simulink model "IEEE14_case"  (R2024b)
settings: Solver=FixedStepAuto  StartTime=0  StopTime=2  FixedStep=1e-7  RelTol=1e-3
values from neighbouring files (symbols this model uses):
  GFL_15_Bva = 0.009    [IEEE14_parameters.m]
  GFL_15_C_bus_pu = 7.179419    [IEEE14_parameters.m]
  GFL_15_f0 = 60    [IEEE14_parameters.m]
  GFL_15_I_id = 691.26967    [IEEE14_parameters.m]
  GFL_15_I_iq = 691.26967    [IEEE14_parameters.m]
  GFL_15_I_od = 45.2207    [IEEE14_parameters.m]
  GFL_15_I_oq = 45.2207    [IEEE14_parameters.m]
  GFL_15_I_pll = 0.78    [IEEE14_parameters.m]
  GFL_15_Kdi = 0.09    [IEEE14_parameters.m]
  GFL_15_Kdo = 0.9    [IEEE14_parameters.m]
  GFL_15_Kqi = 0.09    [IEEE14_parameters.m]
  GFL_15_Kqo = 0.9    [IEEE14_parameters.m]
  GFL_15_Lg_pu = 0.631447    [IEEE14_parameters.m]
  GFL_15_mode = 1    [IEEE14_parameters.m]
  GFL_15_P_id = 3.7166    [IEEE14_parameters.m]
  GFL_15_P_iq = 3.7166    [IEEE14_parameters.m]
  GFL_15_P_od = 0.4798    [IEEE14_parameters.m]
  GFL_15_P_oq = 0.4798    [IEEE14_parameters.m]
  GFL_15_P_pll = 290.42    [IEEE14_parameters.m]
  GFL_15_Qe_ref = 0.2    [IEEE14_parameters.m]
  GFL_15_Rg_pu = 0.024016    [IEEE14_parameters.m]
  GFL_15_Sbase = 1.000000e+4    (= 10000)    [IEEE14_parameters.m]
  GFL_15_Tdi = 0.01    [IEEE14_parameters.m]
  GFL_15_Tdo = 0.2    [IEEE14_parameters.m]
  GFL_15_Tqi = 0.01    [IEEE14_parameters.m]
  GFL_15_Tqo = 0.2    [IEEE14_parameters.m]
  GFL_15_Vbase = 380    [IEEE14_parameters.m]
  GFL_15_Vdc_ref = 1.011475    [IEEE14_parameters.m]
  GFL_15_Vdcbase = 700    [IEEE14_parameters.m]
  GFL_15_vq_ref = 0    [IEEE14_parameters.m]
  GFL_16_Bva = 0.002    [IEEE14_parameters.m]
  GFL_16_C_bus_pu = 7.179419    [IEEE14_parameters.m]
  GFL_16_f0 = 60    [IEEE14_parameters.m]
  GFL_16_I_id = 691.26967    [IEEE14_parameters.m]
  GFL_16_I_iq = 691.26967    [IEEE14_parameters.m]
  GFL_16_I_od = 45.2207    [IEEE14_parameters.m]
  GFL_16_I_oq = 45.2207    [IEEE14_parameters.m]
  GFL_16_I_pll = 0.78    [IEEE14_parameters.m]
  GFL_16_Kdi = 0.05    [IEEE14_parameters.m]
  GFL_16_Kdo = 0.5    [IEEE14_parameters.m]
  GFL_16_Kqi = 0.05    [IEEE14_parameters.m]
  GFL_16_Kqo = 0.5    [IEEE14_parameters.m]
  GFL_16_Lg_pu = 0.631447    [IEEE14_parameters.m]
  GFL_16_mode = 1    [IEEE14_parameters.m]
  GFL_16_P_id = 3.7166    [IEEE14_parameters.m]
  GFL_16_P_iq = 3.7166    [IEEE14_parameters.m]
  GFL_16_P_od = 0.4798    [IEEE14_parameters.m]
  GFL_16_P_oq = 0.4798    [IEEE14_parameters.m]
  GFL_16_P_pll = 290.42    [IEEE14_parameters.m]
  GFL_16_Qe_ref = 0.2    [IEEE14_parameters.m]
  GFL_16_Rg_pu = 0.024016    [IEEE14_parameters.m]
  GFL_16_Sbase = 1.000000e+4    (= 10000)    [IEEE14_parameters.m]
  GFL_16_Tdi = 0.01    [IEEE14_parameters.m]
  GFL_16_Tdo = 0.2    [IEEE14_parameters.m]
  GFL_16_Tqi = 0.01    [IEEE14_parameters.m]
  GFL_16_Tqo = 0.2    [IEEE14_parameters.m]
  GFL_16_Vbase = 380    [IEEE14_parameters.m]
  GFL_16_Vdc_ref = 1.01144    [IEEE14_parameters.m]
  GFL_16_Vdcbase = 700    [IEEE14_parameters.m]
  GFL_16_vq_ref = 0    [IEEE14_parameters.m]
  GFL_17_Bva = 0.002    [IEEE14_parameters.m]
  GFL_17_C_bus_pu = 7.179419    [IEEE14_parameters.m]
  GFL_17_f0 = 60    [IEEE14_parameters.m]
  GFL_17_I_id = 691.26967    [IEEE14_parameters.m]
  GFL_17_I_iq = 691.26967    [IEEE14_parameters.m]
  GFL_17_I_od = 45.2207    [IEEE14_parameters.m]
  GFL_17_I_oq = 45.2207    [IEEE14_parameters.m]
  GFL_17_I_pll = 0.78    [IEEE14_parameters.m]
  GFL_17_Kdi = 0.05    [IEEE14_parameters.m]
  GFL_17_Kdo = 0.5    [IEEE14_parameters.m]
  GFL_17_Kqi = 0.05    [IEEE14_parameters.m]
  GFL_17_Kqo = 0.5    [IEEE14_parameters.m]
  GFL_17_Lg_pu = 0.631447    [IEEE14_parameters.m]
  GFL_17_mode = 1    [IEEE14_parameters.m]
  GFL_17_P_id = 3.7166    [IEEE14_parameters.m]
  GFL_17_P_iq = 3.7166    [IEEE14_parameters.m]
  GFL_17_P_od = 0.4798    [IEEE14_parameters.m]
  GFL_17_P_oq = 0.4798    [IEEE14_parameters.m]
  GFL_17_P_pll = 290.42    [IEEE14_parameters.m]
  GFL_17_Qe_ref = 0.2    [IEEE14_parameters.m]
  GFL_17_Rg_pu = 0.024016    [IEEE14_parameters.m]
  GFL_17_Sbase = 1.000000e+4    (= 10000)    [IEEE14_parameters.m]
  GFL_17_Tdi = 0.01    [IEEE14_parameters.m]
  GFL_17_Tdo = 0.2    [IEEE14_parameters.m]
  GFL_17_Tqi = 0.01    [IEEE14_parameters.m]
  GFL_17_Tqo = 0.2    [IEEE14_parameters.m]
  GFL_17_Vbase = 380    [IEEE14_parameters.m]
  GFL_17_Vdc_ref = 1.011632    [IEEE14_parameters.m]
  GFL_17_Vdcbase = 700    [IEEE14_parameters.m]
  GFL_17_vq_ref = 0    [IEEE14_parameters.m]
  GFL_18_Bva = 0.002    [IEEE14_parameters.m]
  GFL_18_C_bus_pu = 7.179419    [IEEE14_parameters.m]
  GFL_18_f0 = 60    [IEEE14_parameters.m]
  GFL_18_I_id = 691.26967    [IEEE14_parameters.m]
  GFL_18_I_iq = 691.26967    [IEEE14_parameters.m]
  GFL_18_I_od = 45.2207    [IEEE14_parameters.m]
  GFL_18_I_oq = 45.2207    [IEEE14_parameters.m]
  GFL_18_I_pll = 0.78    [IEEE14_parameters.m]
  GFL_18_Kdi = 0.05    [IEEE14_parameters.m]
  GFL_18_Kdo = 0.5    [IEEE14_parameters.m]
  GFL_18_Kqi = 0.05    [IEEE14_parameters.m]
  GFL_18_Kqo = 0.5    [IEEE14_parameters.m]
  GFL_18_Lg_pu = 0.631447    [IEEE14_parameters.m]
  GFL_18_mode = 1    [IEEE14_parameters.m]
  GFL_18_P_id = 3.7166    [IEEE14_parameters.m]
  GFL_18_P_iq = 3.7166    [IEEE14_parameters.m]
  GFL_18_P_od = 0.4798    [IEEE14_parameters.m]
  GFL_18_P_oq = 0.4798    [IEEE14_parameters.m]
  GFL_18_P_pll = 290.42    [IEEE14_parameters.m]
  GFL_18_Qe_ref = 0.2    [IEEE14_parameters.m]
  GFL_18_Rg_pu = 0.024016    [IEEE14_parameters.m]
  GFL_18_Sbase = 1.000000e+4    (= 10000)    [IEEE14_parameters.m]
  GFL_18_Tdi = 0.01    [IEEE14_parameters.m]
  GFL_18_Tdo = 0.2    [IEEE14_parameters.m]
  GFL_18_Tqi = 0.01    [IEEE14_parameters.m]
  GFL_18_Tqo = 0.2    [IEEE14_parameters.m]
  GFL_18_Vbase = 380    [IEEE14_parameters.m]
  GFL_18_Vdc_ref = 1.011572    [IEEE14_parameters.m]
  GFL_18_Vdcbase = 700    [IEEE14_parameters.m]
  GFL_18_vq_ref = 0    [IEEE14_parameters.m]
  ... (+180 more)
(part 15 of 25)

== system IEEE14_case/GFL_18/d_i_gq_GFL_18_block ==
  note: d_i_gq_GFL_18 in case14gfl
      | $\frac{2\,\pi \,\mathrm{Sbase}\,f_{0}\,\left(\Phi _{\mathrm{gd},\mathrm{GFL},18}+P_{\mathrm{iq}}\,\left(\mathrm{Iqv}_{\mathrm{GFL},18}+\Phi _{\mathrm{gc},\mathrm{GFL},18}-i_{\mathrm{gq},\mathrm{GFL},18}-P_{\mathrm{oq}}\,\left(\mathrm{Qe}_{\mathrm{ref}}\,\mathrm{Sbase}+1.73205080756888\,\mathrm{Vbase}\,i_{\mathrm{gd},\mathrm{GFL},18}\,\left(v_{q,\mathrm{GFL},18}\,\cos\left(\theta _{\mathrm{pll},\mathrm{GFL},18}\right)+v_{d,\mathrm{GFL},18}\,\sin\left(\theta _{\mathrm{pll},\mathrm{GFL},18}\right)\right)+1.73205080756888\,\mathrm{Vbase}\,i_{\mathrm{gq},\mathrm{GFL},18}\,\left(v_{d,\mathrm{GFL},18}\,\cos\left(\theta _{\mathrm{pll},\mathrm{GFL},18}\right)-v_{q,\mathrm{GFL},18}\,\sin\left(\theta _{\mathrm{pll},\mathrm{GFL},18}\right)\right)\right)+\mathrm{Bva}\,\mathrm{Vbase}\,\left(v_{q,\mathrm{GFL},18}\,\cos\left(\theta _{\mathrm{pll},\mathrm{GFL},18}\right)+v_{d,\mathrm{GFL},18}\,\sin\left(\theta _{\mathrm{pll},\mathrm{GFL},18}\right)\right)\right)-\frac{\mathrm{Rg}_{\mathrm{pu}}\,{\mathrm{Vbase}}^2\,i_{\mathrm{gq},\mathrm{GFL},18}}{\mathrm{Sbase}}\right)}{\mathrm{Lg}_{\mathrm{pu}}\,{\mathrm{Vbase}}^2}$
      | Automatically generated on 2025-10-09 21:37:31 .
  Input_v_d_GFL_18_6f882 : Inport
  State_theta_pll_GFL_18_750f2 : Inport  Port=2
  Input_v_q_GFL_18_fb235 : Inport  Port=3
  State_theta_pll_GFL_18_9acfa : Inport  Port=4
  State_Iqv_GFL_18_30b1b : Inport  Port=5
  State_i_gd_GFL_18_52805 : Inport  Port=6
  Input_v_d_GFL_18_7a2d9 : Inport  Port=7
  State_theta_pll_GFL_18_d5076 : Inport  Port=8
  Input_v_q_GFL_18_2227f : Inport  Port=9
  State_theta_pll_GFL_18_46ba7 : Inport  Port=10
  State_i_gq_GFL_18_16534 : Inport  Port=11
  Input_v_d_GFL_18_2cf8e : Inport  Port=12
  State_theta_pll_GFL_18_ab8d9 : Inport  Port=13
  Input_v_q_GFL_18_563cc : Inport  Port=14
  State_theta_pll_GFL_18_cabe0 : Inport  Port=15
  State_Phi_gc_GFL_18_55584 : Inport  Port=16
  State_i_gq_GFL_18_9395d : Inport  Port=17
  State_Phi_gd_GFL_18_5fde0 : Inport  Port=18
  State_i_gq_GFL_18_b9a26 : Inport  Port=19
  Add_02e4d : Sum
  Add_19415 : Sum
  Add_1cbed : Sum
  Add_3289e : Sum
  Add_8a5df : Sum
  Add_efdee : Sum
  Constant_-1_893c0 : Constant  Value=-1
  Constant_1.73205080756888_7f0ab : Constant  Value=1.73205080756888
  Constant_1.73205080756888_dd0c5 : Constant  Value=1.73205080756888
  Constant_2.0_2560d : Constant  Value=2.0
  Constant_2.0_3ecfa : Constant  Value=2.0
  Constant_2.0_c0ff8 : Constant  Value=2.0
  Constant_Bva_65ebe : Constant  Value=Bva
  Constant_Lg_pu_8bb32 : Constant  Value=Lg_pu
  Constant_P_iq_7315b : Constant  Value=P_iq
  Constant_P_oq_2c47f : Constant  Value=P_oq
  Constant_Qe_ref_5f6bf : Constant  Value=Qe_ref
  Constant_Rg_pu_8e3e0 : Constant  Value=Rg_pu
  Constant_Sbase_2f81b : Constant  Value=Sbase
  Constant_Sbase_5e239 : Constant  Value=Sbase
  Constant_Sbase_94de3 : Constant  Value=Sbase
  Constant_Vbase_40973 : Constant  Value=Vbase
  Constant_Vbase_813da : Constant  Value=Vbase
  Constant_Vbase_8fd64 : Constant  Value=Vbase
  Constant_Vbase_ae26f : Constant  Value=Vbase
  Constant_Vbase_dbf74 : Constant  Value=Vbase
  Constant_f0_0d82f : Constant  Value=f0
  Constant_pi_8b980 : Constant  Value=pi
  Divide_20004 : Product  Inputs=*/
  Divide_d8df6 : Product  Inputs=*/
  MathFunc_cos_0de55 : Trigonometry  Operator=cos
  MathFunc_cos_104c8 : Trigonometry  Operator=cos
  MathFunc_cos_cc047 : Trigonometry  Operator=cos
  MathFunc_sin_52866 : Trigonometry
  MathFunc_sin_c83ee : Trigonometry
  MathFunc_sin_e5791 : Trigonometry
  Power_7e72b : Math  Operator=pow
  Power_8482d : Math  Operator=pow
  Product_00ff4 : Product
  Product_02cfb : Product
  Product_02fb3 : Product
  Product_04e48 : Product
  Product_17f28 : Product
  Product_1fcf9 : Product
  Product_354b2 : Product
  Product_380b4 : Product
  Product_38262 : Product
  Product_3b5ec : Product
  Product_3c14b : Product
  Product_4982c : Product
  Product_59f52 : Product
  Product_5af2a : Product
  Product_7f0f9 : Product
  Product_8339a : Product
  Product_99a53 : Product
  Product_acf9f : Product
  Product_afc64 : Product
  Product_b291c : Product
  Product_cbf79 : Product
  Product_ebe1d : Product
  Product_f803d : Product
  Product_fb3b2 : Product
  Product_fdbd3 : Product
  Subtract_3737a : Sum  Inputs=+-
  Subtract_401da : Sum  Inputs=+-
  Subtract_89c9e : Sum  Inputs=+-
  Subtract_e7562 : Sum  Inputs=+-
  Subtract_f2a58 : Sum  Inputs=+-
  Blockout_d_i_gq_GFL_18_699bd : Outport
  wires:
  State_theta_pll_GFL_18_d5076/1 -> MathFunc_sin_52866/1
  Constant_Vbase_ae26f/1 -> Product_38262/2
  State_theta_pll_GFL_18_46ba7/1 -> MathFunc_cos_cc047/1
  Constant_1.73205080756888_dd0c5/1 -> Product_38262/1
  Input_v_d_GFL_18_7a2d9/1 -> Product_3b5ec/1
  MathFunc_sin_52866/1 -> Product_3b5ec/2
  Product_acf9f/1 -> Add_efdee/2
  Input_v_q_GFL_18_2227f/1 -> Product_acf9f/1
  Constant_Sbase_5e239/1 -> Product_380b4/2
  MathFunc_cos_cc047/1 -> Product_acf9f/2
  Constant_Vbase_dbf74/1 -> Product_02fb3/2
  State_theta_pll_GFL_18_ab8d9/1 -> MathFunc_cos_0de55/1
  MathFunc_sin_e5791/1 -> Product_fb3b2/2
  State_theta_pll_GFL_18_cabe0/1 -> MathFunc_sin_e5791/1
  Constant_Qe_ref_5f6bf/1 -> Product_354b2/2
  State_theta_pll_GFL_18_750f2/1 -> MathFunc_sin_c83ee/1
  MathFunc_cos_104c8/1 -> Product_02cfb/2
  State_theta_pll_GFL_18_9acfa/1 -> MathFunc_cos_104c8/1
  Product_354b2/1 -> Product_380b4/1
  Constant_-1_893c0/1 -> Product_354b2/1
  Product_38262/1 -> Product_00ff4/1
  Product_3b5ec/1 -> Add_efdee/1
  State_i_gd_GFL_18_52805/1 -> Product_00ff4/2
  Product_02fb3/1 -> Product_f803d/1
  Constant_1.73205080756888_7f0ab/1 -> Product_02fb3/1
  Product_ebe1d/1 -> Subtract_f2a58/1
  Input_v_d_GFL_18_2cf8e/1 -> Product_ebe1d/1
  MathFunc_cos_0de55/1 -> Product_ebe1d/2
  Product_fb3b2/1 -> Subtract_f2a58/2
  Input_v_q_GFL_18_563cc/1 -> Product_fb3b2/1
  Product_59f52/1 -> Add_02e4d/1
  Input_v_d_GFL_18_6f882/1 -> Product_59f52/1
  MathFunc_sin_c83ee/1 -> Product_59f52/2
  Product_02cfb/1 -> Add_02e4d/2
  Constant_2.0_3ecfa/1 -> Power_7e72b/2
  Input_v_q_GFL_18_fb235/1 -> Product_02cfb/1
  Product_00ff4/1 -> Product_17f28/1
  Add_efdee/1 -> Product_17f28/2
  Subtract_f2a58/1 -> Product_fdbd3/2
  State_i_gq_GFL_18_16534/1 -> Product_f803d/2
  Constant_Sbase_2f81b/1 -> Product_5af2a/2
  Constant_2.0_c0ff8/1 -> Power_8482d/2
  Constant_Bva_65ebe/1 -> Product_7f0f9/1
  Constant_Vbase_8fd64/1 -> Power_8482d/1
  Product_7f0f9/1 -> Product_8339a/1
  Constant_Vbase_40973/1 -> Product_7f0f9/2
  Product_380b4/1 -> Subtract_89c9e/1
  Product_17f28/1 -> Subtract_89c9e/2
  Constant_2.0_2560d/1 -> Product_3c14b/1
  Product_f803d/1 -> Product_fdbd3/1
  Add_02e4d/1 -> Product_8339a/2
  Subtract_89c9e/1 -> Subtract_e7562/1
  Product_cbf79/1 -> Add_3289e/1
  Product_fdbd3/1 -> Subtract_e7562/2
  Power_8482d/1 -> Product_04e48/2
  Product_8339a/1 -> Add_8a5df/1
  Product_afc64/1 -> Add_1cbed/2
  Constant_P_oq_2c47f/1 -> Product_afc64/1
  State_Iqv_GFL_18_30b1b/1 -> Add_8a5df/2
  Subtract_e7562/1 -> Product_afc64/2
  Constant_Rg_pu_8e3e0/1 -> Product_04e48/1
  Add_19415/1 -> Subtract_3737a/1
  Add_8a5df/1 -> Add_1cbed/1
  Add_1cbed/1 -> Add_19415/1
  Product_5af2a/1 -> Product_b291c/1
  State_Phi_gc_GFL_18_55584/1 -> Add_19415/2
  State_i_gq_GFL_18_9395d/1 -> Subtract_3737a/2
  Divide_20004/1 -> Subtract_401da/2
  Constant_pi_8b980/1 -> Product_3c14b/2
  Constant_P_iq_7315b/1 -> Product_cbf79/1
  Subtract_3737a/1 -> Product_cbf79/2
  Product_04e48/1 -> Product_99a53/1
  State_i_gq_GFL_18_b9a26/1 -> Product_99a53/2
  Product_3c14b/1 -> Product_5af2a/1
  State_Phi_gd_GFL_18_5fde0/1 -> Add_3289e/2
  Product_99a53/1 -> Divide_20004/1
  Constant_Sbase_94de3/1 -> Divide_20004/2
  Constant_f0_0d82f/1 -> Product_b291c/2
  Add_3289e/1 -> Subtract_401da/1
  Constant_Vbase_813da/1 -> Power_7e72b/1
  Product_b291c/1 -> Product_4982c/1
  Subtract_401da/1 -> Product_4982c/2
  Constant_Lg_pu_8bb32/1 -> Product_1fcf9/1
  Power_7e72b/1 -> Product_1fcf9/2
  Product_4982c/1 -> Divide_d8df6/1
  Product_1fcf9/1 -> Divide_d8df6/2
  Divide_d8df6/1 -> Blockout_d_i_gq_GFL_18_699bd/1

== system IEEE14_case/GFL_18/d_theta_pll_GFL_18_block ==
  note: d_theta_pll_GFL_18 in case14gfl
      | $\mathrm{Phipll}_{\mathrm{GFL},18}-P_{\mathrm{pll}}\,\left(\mathrm{vq}_{\mathrm{ref}}+v_{q,\mathrm{GFL},18}\,\cos\left(\theta _{\mathrm{pll},\mathrm{GFL},18}\right)+v_{d,\mathrm{GFL},18}\,\sin\left(\theta _{\mathrm{pll},\mathrm{GFL},18}\right)\right)$
      | Automatically generated on 2025-10-09 21:37:47 .
  Input_v_d_GFL_18_139e6 : Inport
  State_theta_pll_GFL_18_5174e : Inport  Port=2
  Input_v_q_GFL_18_f1179 : Inport  Port=3
  State_theta_pll_GFL_18_62af6 : Inport  Port=4
  State_Phipll_GFL_18_8c922 : Inport  Port=5
  Add_b5b31 : Sum
  Constant_-1_efd83 : Constant  Value=-1
  Constant_P_pll_2599c : Constant  Value=P_pll
  Constant_vq_ref_bcbc1 : Constant  Value=vq_ref
  MathFunc_cos_311d9 : Trigonometry  Operator=cos
  MathFunc_sin_30925 : Trigonometry
  Product_14af6 : Product
  Product_73732 : Product
  Product_8c059 : Product
  Product_d04f2 : Product
  Subtract_1f7b4 : Sum  Inputs=+-
  Subtract_b312a : Sum  Inputs=+-
  Blockout_d_theta_pll_GFL_18_8cdeb : Outport
  wires:
  State_theta_pll_GFL_18_62af6/1 -> MathFunc_cos_311d9/1
  MathFunc_cos_311d9/1 -> Product_73732/2
  Product_8c059/1 -> Product_14af6/1
  Input_v_d_GFL_18_139e6/1 -> Product_8c059/2
  Constant_-1_efd83/1 -> Product_8c059/1
  State_theta_pll_GFL_18_5174e/1 -> MathFunc_sin_30925/1
  MathFunc_sin_30925/1 -> Product_14af6/2
  Input_v_q_GFL_18_f1179/1 -> Product_73732/1
  Constant_P_pll_2599c/1 -> Product_d04f2/1
  Constant_vq_ref_bcbc1/1 -> Subtract_b312a/2
  Product_14af6/1 -> Subtract_1f7b4/1
  Subtract_b312a/1 -> Product_d04f2/2
  Product_73732/1 -> Subtract_1f7b4/2
  Subtract_1f7b4/1 -> Subtract_b312a/1
  Product_d04f2/1 -> Add_b5b31/1
  State_Phipll_GFL_18_8c922/1 -> Add_b5b31/2
  Add_b5b31/1 -> Blockout_d_theta_pll_GFL_18_8cdeb/1

== system IEEE14_case/GFL_18/e_dc_GFL_18_block ==
  note: e_dc_GFL_18 in case14gfl
      | $\frac{V_{\mathrm{dc},\mathrm{GFL},18}}{\mathrm{Vdcbase}}$
      | Automatically generated on 2025-10-09 21:38:06 .
  State_V_dc_GFL_18_327dd : Inport
  Constant_Vdcbase_d3a0a : Constant  Value=Vdcbase
  Divide_b057f : Product  Inputs=*/
  Blockout_e_dc_GFL_18_f7b34 : Outport
  wires:
  State_V_dc_GFL_18_327dd/1 -> Divide_b057f/1
  Constant_Vdcbase_d3a0a/1 -> Divide_b057f/2
  Divide_b057f/1 -> Blockout_e_dc_GFL_18_f7b34/1

== system IEEE14_case/GFL_18/i_d_GFL_18_block ==
  note: i_d_GFL_18 in case14gfl
      | $0.00658179306876173\,i_{\mathrm{gd},\mathrm{GFL},18}\,\cos\left(\theta _{\mathrm{pll},\mathrm{GFL},18}\right)+0.00658179306876173\,i_{\mathrm{gq},\mathrm{GFL},18}\,\sin\left(\theta _{\mathrm{pll},\mathrm{GFL},18}\right)$
      | Automatically generated on 2025-10-09 21:38:04 .
  State_i_gd_GFL_18_d192a : Inport
  State_theta_pll_GFL_18_bcee7 : Inport  Port=2
  State_i_gq_GFL_18_5a399 : Inport  Port=3
  State_theta_pll_GFL_18_13217 : Inport  Port=4
  Add_49782 : Sum
  Constant_0.00658179306876173_73b08 : Constant  Value=0.00658179306876173
  Constant_0.00658179306876173_d9046 : Constant  Value=0.00658179306876173
  MathFunc_cos_64f3e : Trigonometry  Operator=cos
  MathFunc_sin_361ad : Trigonometry
  Product_1e23c : Product
  Product_47ac7 : Product
  Product_752ad : Product
  Product_d7e83 : Product
  Blockout_i_d_GFL_18_7425f : Outport
  wires:
  Constant_0.00658179306876173_73b08/1 -> Product_47ac7/1
  Product_47ac7/1 -> Product_752ad/1
  State_i_gd_GFL_18_d192a/1 -> Product_47ac7/2
  State_theta_pll_GFL_18_bcee7/1 -> MathFunc_cos_64f3e/1
  Constant_0.00658179306876173_d9046/1 -> Product_1e23c/1
  State_i_gq_GFL_18_5a399/1 -> Product_1e23c/2
  State_theta_pll_GFL_18_13217/1 -> MathFunc_sin_361ad/1
  MathFunc_cos_64f3e/1 -> Product_752ad/2
  Product_1e23c/1 -> Product_d7e83/1
  MathFunc_sin_361ad/1 -> Product_d7e83/2
  Product_752ad/1 -> Add_49782/1
  Product_d7e83/1 -> Add_49782/2
  Add_49782/1 -> Blockout_i_d_GFL_18_7425f/1

== system IEEE14_case/GFL_18/i_q_GFL_18_block ==
  note: i_q_GFL_18 in case14gfl
      | $0.00658179306876173\,i_{\mathrm{gq},\mathrm{GFL},18}\,\cos\left(\theta _{\mathrm{pll},\mathrm{GFL},18}\right)-0.00658179306876173\,i_{\mathrm{gd},\mathrm{GFL},18}\,\sin\left(\theta _{\mathrm{pll},\mathrm{GFL},18}\right)$
      | Automatically generated on 2025-10-09 21:38:05 .
  State_i_gd_GFL_18_76c93 : Inport
  State_theta_pll_GFL_18_ffcf5 : Inport  Port=2
  State_i_gq_GFL_18_d9fa7 : Inport  Port=3
  State_theta_pll_GFL_18_e08cb : Inport  Port=4
  Add_8dc48 : Sum
  Constant_-0.00658179306876173_03bc6 : Constant  Value=-0.00658179306876173
  Constant_0.00658179306876173_495f2 : Constant  Value=0.00658179306876173
  MathFunc_cos_8264e : Trigonometry  Operator=cos
  MathFunc_sin_8d0e1 : Trigonometry
  Product_0e091 : Product
  Product_75a27 : Product
  Product_7d25d : Product
  Product_c1d13 : Product
  Blockout_i_q_GFL_18_d2cea : Outport
  wires:
  State_i_gd_GFL_18_76c93/1 -> Product_0e091/2
  Constant_-0.00658179306876173_03bc6/1 -> Product_0e091/1
  State_theta_pll_GFL_18_ffcf5/1 -> MathFunc_sin_8d0e1/1
  MathFunc_sin_8d0e1/1 -> Product_7d25d/2
  Product_75a27/1 -> Product_c1d13/1
  Constant_0.00658179306876173_495f2/1 -> Product_75a27/1
  State_i_gq_GFL_18_d9fa7/1 -> Product_75a27/2
  MathFunc_cos_8264e/1 -> Product_c1d13/2
  State_theta_pll_GFL_18_e08cb/1 -> MathFunc_cos_8264e/1
  Product_0e091/1 -> Product_7d25d/1
  Product_7d25d/1 -> Add_8dc48/1
  Product_c1d13/1 -> Add_8dc48/2
  Add_8dc48/1 -> Blockout_i_q_GFL_18_d2cea/1

== system IEEE14_case/SG_D_1/T_e_SG_D_1_block ==
  note: T_e_SG_D_1 in case14gfl
      | $-\frac{\psi _{d,\mathrm{SG},D,1}\,\left(\psi _{q,\mathrm{SG},D,1}+\frac{\psi _{\mathrm{gq},\mathrm{SG},D,1}\,\left(x_{l}-x_{\mathrm{qdd}}\right)}{x_{l}-x_{\mathrm{qd}}}+\frac{\psi _{\mathrm{kq},\mathrm{SG},D,1}\,\left(x_{\mathrm{qd}}-x_{\mathrm{qdd}}\right)}{x_{l}-x_{\mathrm{qd}}}\right)}{x_{\mathrm{qdd}}}-\frac{\psi _{q,\mathrm{SG},D,1}\,\left(\frac{\psi _{\mathrm{1d},\mathrm{SG},D,1}\,\left(x_{\mathrm{dd}}-x_{\mathrm{ddd}}\right)}{x_{\mathrm{dd}}-x_{l}}-\psi _{d,\mathrm{SG},D,1}+\frac{\psi _{\mathrm{fd},\mathrm{SG},D,1}\,\left(x_{\mathrm{ddd}}-x_{l}\right)}{x_{\mathrm{dd}}-x_{l}}\right)}{x_{\mathrm{ddd}}}$
      | Automatically generated on 2025-10-09 21:30:38 .
  State_psi_d_SG_D_1_5a569 : Inport
  State_psi_gq_SG_D_1_b91dd : Inport  Port=2
  State_psi_kq_SG_D_1_246e1 : Inport  Port=3
  State_psi_q_SG_D_1_fd30f : Inport  Port=4
  State_psi_q_SG_D_1_04e42 : Inport  Port=5
  State_psi_1d_SG_D_1_ba9b8 : Inport  Port=6
  State_psi_d_SG_D_1_dfbb8 : Inport  Port=7
  State_psi_fd_SG_D_1_a5ec6 : Inport  Port=8
  Add_15813 : Sum
  Add_52817 : Sum
  Add_5c53b : Sum
  Add_888d1 : Sum
  Add_e87b4 : Sum
  Add_faa3f : Sum
  Constant_-1_20ebd : Constant  Value=-1
  Constant_-1_23088 : Constant  Value=-1
  Constant_-1_5c44f : Constant  Value=-1
  Constant_-1_7ef1e : Constant  Value=-1
  Constant_-1_819bd : Constant  Value=-1
  Constant_x_dd_afa26 : Constant  Value=x_dd
  Constant_x_dd_bbb31 : Constant  Value=x_dd
  Constant_x_dd_ef5d8 : Constant  Value=x_dd
  Constant_x_ddd_5c83e : Constant  Value=x_ddd
  Constant_x_ddd_9041a : Constant  Value=x_ddd
  Constant_x_ddd_9558c : Constant  Value=x_ddd
  Constant_x_l_0264b : Constant  Value=x_l
  Constant_x_l_11835 : Constant  Value=x_l
  Constant_x_l_11c0c : Constant  Value=x_l
  Constant_x_l_236bd : Constant  Value=x_l
  Constant_x_l_af79b : Constant  Value=x_l
  Constant_x_l_d29d0 : Constant  Value=x_l
  Constant_x_qd_00b16 : Constant  Value=x_qd
  Constant_x_qd_65a83 : Constant  Value=x_qd
  Constant_x_qd_a36f6 : Constant  Value=x_qd
  Constant_x_qdd_3a7f8 : Constant  Value=x_qdd
  Constant_x_qdd_6fb1f : Constant  Value=x_qdd
  Constant_x_qdd_7f14f : Constant  Value=x_qdd
  Divide_3372a : Product  Inputs=*/
  Divide_4141f : Product  Inputs=*/
  Divide_a977c : Product  Inputs=*/
  Divide_b2e43 : Product  Inputs=*/
  Divide_c6934 : Product  Inputs=*/
  Divide_e1df0 : Product  Inputs=*/
  Product_03874 : Product
  Product_296a6 : Product
  Product_3b462 : Product
  Product_45542 : Product
  Product_48980 : Product
  Product_48ca3 : Product
  Product_6ef4a : Product
  Product_791c2 : Product
  Product_9bd06 : Product
  Product_cbf80 : Product
  Product_ff354 : Product
  Subtract_0b243 : Sum  Inputs=+-
  Subtract_187e6 : Sum  Inputs=+-
  Subtract_54017 : Sum  Inputs=+-
  Subtract_97566 : Sum  Inputs=+-
  Subtract_9d862 : Sum  Inputs=+-
  Subtract_d3fe2 : Sum  Inputs=+-
  Subtract_e157c : Sum  Inputs=+-
  Blockout_T_e_SG_D_1_52337 : Outport
  wires:
  Product_296a6/1 -> Divide_b2e43/1
  Product_45542/1 -> Add_888d1/1
  Divide_b2e43/1 -> Subtract_187e6/1
  Constant_-1_7ef1e/1 -> Product_45542/1
  Constant_x_l_11835/1 -> Product_45542/2
  Constant_x_qdd_7f14f/1 -> Add_888d1/2
  Constant_x_qd_a36f6/1 -> Subtract_97566/1
  Constant_-1_23088/1 -> Product_48ca3/1
  Constant_x_qdd_6fb1f/1 -> Divide_3372a/2
  Constant_x_qdd_3a7f8/1 -> Subtract_97566/2
  State_psi_q_SG_D_1_04e42/1 -> Product_cbf80/1
  Constant_x_dd_ef5d8/1 -> Subtract_0b243/1
  Constant_x_l_236bd/1 -> Product_48ca3/2
  Subtract_0b243/1 -> Product_03874/2
  Constant_-1_819bd/1 -> Product_791c2/1
  Constant_x_l_d29d0/1 -> Product_791c2/2
  Subtract_9d862/1 -> Product_cbf80/2
  State_psi_q_SG_D_1_fd30f/1 -> Add_52817/2
  Constant_-1_5c44f/1 -> Product_9bd06/1
  State_psi_1d_SG_D_1_ba9b8/1 -> Product_9bd06/2
  Constant_x_ddd_5c83e/1 -> Subtract_0b243/2
  State_psi_gq_SG_D_1_b91dd/1 -> Product_296a6/1
  Add_888d1/1 -> Product_296a6/2
  Product_48ca3/1 -> Add_5c53b/1
  Product_3b462/1 -> Product_ff354/1
  Constant_x_qd_65a83/1 -> Add_5c53b/2
  Product_03874/1 -> Divide_c6934/1
  State_psi_kq_SG_D_1_246e1/1 -> Product_6ef4a/1
  Add_5c53b/1 -> Divide_b2e43/2
  Subtract_97566/1 -> Product_6ef4a/2
  Product_791c2/1 -> Add_e87b4/1
  Constant_x_qd_00b16/1 -> Add_e87b4/2
  Product_6ef4a/1 -> Divide_e1df0/1
  Product_9bd06/1 -> Product_03874/1
  Constant_x_dd_afa26/1 -> Subtract_54017/1
  Constant_x_l_af79b/1 -> Subtract_54017/2
  Constant_x_ddd_9558c/1 -> Subtract_e157c/1
  Product_cbf80/1 -> Divide_a977c/1
  Constant_x_l_11c0c/1 -> Subtract_e157c/2
  Divide_3372a/1 -> Add_15813/1
  Product_ff354/1 -> Divide_3372a/1
  Add_e87b4/1 -> Divide_e1df0/2
  Subtract_187e6/1 -> Add_52817/1
  Divide_e1df0/1 -> Subtract_187e6/2
  Subtract_54017/1 -> Divide_c6934/2
  State_psi_fd_SG_D_1_a5ec6/1 -> Product_48980/1
  Constant_x_ddd_9041a/1 -> Divide_a977c/2
  Subtract_e157c/1 -> Product_48980/2
  Constant_x_dd_bbb31/1 -> Subtract_d3fe2/1
  Constant_x_l_0264b/1 -> Subtract_d3fe2/2
  Divide_c6934/1 -> Add_faa3f/1
  Add_faa3f/1 -> Subtract_9d862/1
  State_psi_d_SG_D_1_dfbb8/1 -> Add_faa3f/2
  Product_48980/1 -> Divide_4141f/1
  Subtract_d3fe2/1 -> Divide_4141f/2
  Constant_-1_20ebd/1 -> Product_3b462/1
  State_psi_d_SG_D_1_5a569/1 -> Product_3b462/2
  Divide_4141f/1 -> Subtract_9d862/2
  Add_52817/1 -> Product_ff354/2
  Divide_a977c/1 -> Add_15813/2
  Add_15813/1 -> Blockout_T_e_SG_D_1_52337/1

== system IEEE14_case/SG_D_1/d_E_fd_SG_D_1_block ==
  note: d_E_fd_SG_D_1 in case14gfl
      | $\frac{V_{f,\mathrm{SG},D,1}-E_{\mathrm{fd},\mathrm{SG},D,1}\,K_{E}}{T_{E}}$
      | Automatically generated on 2025-10-09 21:30:23 .
  State_E_fd_SG_D_1_314b1 : Inport
  State_V_f_SG_D_1_aa35b : Inport  Port=2
  Add_7efa5 : Sum
  Constant_-1_280cb : Constant  Value=-1
  Constant_K_E_b5908 : Constant  Value=K_E
  Constant_T_E_8fc46 : Constant  Value=T_E
  Divide_5b867 : Product  Inputs=*/
  Product_9f6cd : Product
  Product_cf6f3 : Product
  Blockout_d_E_fd_SG_D_1_7b54f : Outport
  wires:
  Add_7efa5/1 -> Divide_5b867/1
  Constant_-1_280cb/1 -> Product_9f6cd/1
  State_E_fd_SG_D_1_314b1/1 -> Product_9f6cd/2
  Product_9f6cd/1 -> Product_cf6f3/1
  Constant_K_E_b5908/1 -> Product_cf6f3/2
  Product_cf6f3/1 -> Add_7efa5/1
  Constant_T_E_8fc46/1 -> Divide_5b867/2
  State_V_f_SG_D_1_aa35b/1 -> Add_7efa5/2
  Divide_5b867/1 -> Blockout_d_E_fd_SG_D_1_7b54f/1

== system IEEE14_case/SG_D_1/d_Px_1_SG_D_1_block ==
  note: d_Px_1_SG_D_1 in case14gfl
      | $\frac{w_{\mathrm{SG},D,1}-2\,\pi \,f_{0}}{T_{w}}-\frac{\mathrm{Px}_{1,\mathrm{SG},D,1}}{T_{w}}$
      | Automatically generated on 2025-10-09 21:30:24 .
  State_Px_1_SG_D_1_41b99 : Inport
  State_w_SG_D_1_183d0 : Inport  Port=2
  Add_88c60 : Sum
  Add_cdc76 : Sum
  Constant_-1_b4f57 : Constant  Value=-1
  Constant_-2.0_fceb0 : Constant  Value=-2.0
  Constant_T_w_684c9 : Constant  Value=T_w
  Constant_T_w_880fd : Constant  Value=T_w
  Constant_f0_24278 : Constant  Value=f0
  Constant_pi_74ff2 : Constant  Value=pi
  Divide_2bf1d : Product  Inputs=*/
  Divide_a90f1 : Product  Inputs=*/
  Product_51726 : Product
  Product_ac4ab : Product
  Product_c92ab : Product
  Blockout_d_Px_1_SG_D_1_a4a61 : Outport
  wires:
  Add_88c60/1 -> Blockout_d_Px_1_SG_D_1_a4a61/1
  Constant_-2.0_fceb0/1 -> Product_51726/1
  Product_ac4ab/1 -> Divide_2bf1d/1
  State_w_SG_D_1_183d0/1 -> Add_cdc76/2
  Constant_-1_b4f57/1 -> Product_ac4ab/1
  Constant_f0_24278/1 -> Product_c92ab/2
  Constant_pi_74ff2/1 -> Product_51726/2
  Product_c92ab/1 -> Add_cdc76/1
  Product_51726/1 -> Product_c92ab/1
  State_Px_1_SG_D_1_41b99/1 -> Product_ac4ab/2
  Constant_T_w_684c9/1 -> Divide_2bf1d/2
  Add_cdc76/1 -> Divide_a90f1/1
  Constant_T_w_880fd/1 -> Divide_a90f1/2
  Divide_2bf1d/1 -> Add_88c60/1
  Divide_a90f1/1 -> Add_88c60/2

== system IEEE14_case/SG_D_1/d_Px_2_SG_D_1_block ==
  note: d_Px_2_SG_D_1 in case14gfl
      | $\frac{\mathrm{Px}_{1,\mathrm{SG},D,1}-T_{2}\,\left(\frac{\mathrm{Px}_{1,\mathrm{SG},D,1}}{T_{w}}-\frac{w_{\mathrm{SG},D,1}-2\,\pi \,f_{0}}{T_{w}}\right)}{T_{1}}-\frac{\mathrm{Px}_{2,\mathrm{SG},D,1}}{T_{1}}$
      | Automatically generated on 2025-10-09 21:30:25 .
  State_Px_2_SG_D_1_52166 : Inport
  State_Px_1_SG_D_1_02194 : Inport  Port=2
  State_Px_1_SG_D_1_ca7d0 : Inport  Port=3
  State_w_SG_D_1_83c31 : Inport  Port=4
  Add_5c313 : Sum
  Add_d1ec7 : Sum
  Add_e70f9 : Sum
  Add_ed887 : Sum
  Constant_-1_8b1aa : Constant  Value=-1
  Constant_-1_efaad : Constant  Value=-1
  Constant_-2.0_92cd5 : Constant  Value=-2.0
  Constant_T_1_1e374 : Constant  Value=T_1
  Constant_T_1_8a9e7 : Constant  Value=T_1
  Constant_T_2_95950 : Constant  Value=T_2
  Constant_T_w_8aedd : Constant  Value=T_w
  Constant_T_w_9a58d : Constant  Value=T_w
  Constant_f0_6a979 : Constant  Value=f0
  Constant_pi_69901 : Constant  Value=pi
  Divide_24880 : Product  Inputs=*/
  Divide_59b60 : Product  Inputs=*/
  Divide_5ee69 : Product  Inputs=*/
  Divide_cfcd7 : Product  Inputs=*/
  Product_1799e : Product
  Product_1aa52 : Product
  Product_4a613 : Product
  Product_77749 : Product
  Product_f0c2a : Product
  Blockout_d_Px_2_SG_D_1_c2665 : Outport
  wires:
  Constant_-2.0_92cd5/1 -> Product_f0c2a/1
  State_w_SG_D_1_83c31/1 -> Add_ed887/2
  Constant_f0_6a979/1 -> Product_77749/2
  Constant_pi_69901/1 -> Product_f0c2a/2
  Add_d1ec7/1 -> Product_1aa52/2
  Product_77749/1 -> Add_ed887/1
  Divide_59b60/1 -> Add_d1ec7/1
  Product_f0c2a/1 -> Product_77749/1
  Constant_T_w_8aedd/1 -> Divide_59b60/2
  Constant_-1_8b1aa/1 -> Product_4a613/1
  State_Px_1_SG_D_1_ca7d0/1 -> Product_4a613/2
  Divide_cfcd7/1 -> Add_5c313/1
  Product_4a613/1 -> Divide_59b60/1
  Add_ed887/1 -> Divide_24880/1
  Constant_T_w_9a58d/1 -> Divide_24880/2
  Divide_24880/1 -> Add_d1ec7/2
  Constant_T_2_95950/1 -> Product_1aa52/1
  Constant_-1_efaad/1 -> Product_1799e/1
  State_Px_2_SG_D_1_52166/1 -> Product_1799e/2
  State_Px_1_SG_D_1_02194/1 -> Add_e70f9/1
  Product_1aa52/1 -> Add_e70f9/2
  Add_e70f9/1 -> Divide_5ee69/1
  Product_1799e/1 -> Divide_cfcd7/1
  Constant_T_1_1e374/1 -> Divide_cfcd7/2
  Constant_T_1_8a9e7/1 -> Divide_5ee69/2
  Divide_5ee69/1 -> Add_5c313/2
  Add_5c313/1 -> Blockout_d_Px_2_SG_D_1_c2665/1

== system IEEE14_case/SG_D_1/d_Px_3_SG_D_1_block ==
  note: d_Px_3_SG_D_1 in case14gfl
      | $\frac{\mathrm{Px}_{2,\mathrm{SG},D,1}+T_{4}\,\left(\frac{\mathrm{Px}_{1,\mathrm{SG},D,1}-T_{2}\,\left(\frac{\mathrm{Px}_{1,\mathrm{SG},D,1}}{T_{w}}-\frac{w_{\mathrm{SG},D,1}-2\,\pi \,f_{0}}{T_{w}}\right)}{T_{1}}-\frac{\mathrm{Px}_{2,\mathrm{SG},D,1}}{T_{1}}\right)}{T_{3}}-\frac{\mathrm{Px}_{3,\mathrm{SG},D,1}}{T_{3}}$
      | Automatically generated on 2025-10-09 21:30:27 .
  State_Px_3_SG_D_1_65e83 : Inport
  State_Px_2_SG_D_1_173b9 : Inport  Port=2
  State_Px_2_SG_D_1_5b4c4 : Inport  Port=3
  State_Px_1_SG_D_1_d599f : Inport  Port=4
  State_Px_1_SG_D_1_5257c : Inport  Port=5
  State_w_SG_D_1_d6c43 : Inport  Port=6
  Add_232e9 : Sum
  Add_25541 : Sum
  Add_4762f : Sum
  Add_58032 : Sum
  Add_68405 : Sum
  Add_8004e : Sum
  Constant_-1_16cf1 : Constant  Value=-1
  Constant_-1_c7b08 : Constant  Value=-1
  Constant_-1_dff9a : Constant  Value=-1
  Constant_-2.0_b0ca5 : Constant  Value=-2.0
  Constant_T_1_7939c : Constant  Value=T_1
  Constant_T_1_f62f1 : Constant  Value=T_1
  Constant_T_2_bb48c : Constant  Value=T_2
  Constant_T_3_62f6c : Constant  Value=T_3
  Constant_T_3_74862 : Constant  Value=T_3
  Constant_T_4_db4d0 : Constant  Value=T_4
  Constant_T_w_02c5f : Constant  Value=T_w
  Constant_T_w_cb87b : Constant  Value=T_w
  Constant_f0_aa80e : Constant  Value=f0
  Constant_pi_ac92a : Constant  Value=pi
  Divide_898d9 : Product  Inputs=*/
  Divide_89b0c : Product  Inputs=*/
  Divide_91f73 : Product  Inputs=*/
  Divide_b839b : Product  Inputs=*/
  Divide_c42a8 : Product  Inputs=*/
  Divide_e9b75 : Product  Inputs=*/
  Product_36988 : Product
  Product_37d02 : Product
  Product_3d2a3 : Product
  Product_6adc6 : Product
  Product_bbfcc : Product
  Product_c627f : Product
  Product_cfaa7 : Product
  Blockout_d_Px_3_SG_D_1_27eea : Outport
  wires:
  Constant_T_w_cb87b/1 -> Divide_91f73/2
  Constant_-1_dff9a/1 -> Product_3d2a3/1
  Add_8004e/1 -> Blockout_d_Px_3_SG_D_1_27eea/1
  Constant_-2.0_b0ca5/1 -> Product_37d02/1
  State_w_SG_D_1_d6c43/1 -> Add_58032/2
  Constant_f0_aa80e/1 -> Product_c627f/2
  State_Px_1_SG_D_1_5257c/1 -> Product_3d2a3/2
  Constant_pi_ac92a/1 -> Product_37d02/2
  Product_c627f/1 -> Add_58032/1
  Product_37d02/1 -> Product_c627f/1
  Product_3d2a3/1 -> Divide_91f73/1
  Divide_898d9/1 -> Add_8004e/1
  Constant_T_3_74862/1 -> Divide_b839b/2
  Add_58032/1 -> Divide_c42a8/1
  Constant_T_w_02c5f/1 -> Divide_c42a8/2
  Divide_91f73/1 -> Add_232e9/1
  Divide_c42a8/1 -> Add_232e9/2
  Constant_-1_16cf1/1 -> Product_36988/1
  Constant_T_2_bb48c/1 -> Product_bbfcc/1
  Add_232e9/1 -> Product_bbfcc/2
  Constant_-1_c7b08/1 -> Product_cfaa7/1
  Divide_b839b/1 -> Add_8004e/2
  Constant_T_3_62f6c/1 -> Divide_898d9/2
  State_Px_2_SG_D_1_5b4c4/1 -> Product_cfaa7/2
  State_Px_1_SG_D_1_d599f/1 -> Add_4762f/1
  Divide_e9b75/1 -> Add_68405/1
  Product_bbfcc/1 -> Add_4762f/2
  Product_cfaa7/1 -> Divide_e9b75/1
  Product_36988/1 -> Divide_898d9/1
  Constant_T_1_f62f1/1 -> Divide_e9b75/2
  Add_4762f/1 -> Divide_89b0c/1
  Constant_T_1_7939c/1 -> Divide_89b0c/2
  Divide_89b0c/1 -> Add_68405/2
  Constant_T_4_db4d0/1 -> Product_6adc6/1
  Add_68405/1 -> Product_6adc6/2
  State_Px_3_SG_D_1_65e83/1 -> Product_36988/2
  State_Px_2_SG_D_1_173b9/1 -> Add_25541/1
  Product_6adc6/1 -> Add_25541/2
  Add_25541/1 -> Divide_b839b/1

== system IEEE14_case/SG_D_1/d_R_f_SG_D_1_block ==
  note: d_R_f_SG_D_1 in case14gfl
      | $-\frac{R_{f,\mathrm{SG},D,1}-\frac{E_{\mathrm{fd},\mathrm{SG},D,1}\,K_{F}}{T_{F}}}{T_{F}}$
      | Automatically generated on 2025-10-09 21:30:22 .
  State_E_fd_SG_D_1_43088 : Inport
  State_R_f_SG_D_1_c9358 : Inport  Port=2
  Constant_K_F_b9c01 : Constant  Value=K_F
  Constant_T_F_36063 : Constant  Value=T_F
  Constant_T_F_36415 : Constant  Value=T_F
  Divide_d5eef : Product  Inputs=*/
  Divide_e270d : Product  Inputs=*/
  Product_43e0c : Product
  Subtract_ec892 : Sum  Inputs=+-
  Blockout_d_R_f_SG_D_1_dc367 : Outport
  wires:
  Constant_K_F_b9c01/1 -> Product_43e0c/2
  Product_43e0c/1 -> Divide_d5eef/1
  State_E_fd_SG_D_1_43088/1 -> Product_43e0c/1
  State_R_f_SG_D_1_c9358/1 -> Subtract_ec892/2
  Constant_T_F_36063/1 -> Divide_d5eef/2
  Divide_d5eef/1 -> Subtract_ec892/1
  Divide_e270d/1 -> Blockout_d_R_f_SG_D_1_dc367/1
  Subtract_ec892/1 -> Divide_e270d/1
  Constant_T_F_36415/1 -> Divide_e270d/2

== system IEEE14_case/SG_D_1/d_T_m_SG_D_1_block ==
  note: d_T_m_SG_D_1 in case14gfl
      | $-\frac{T_{m,\mathrm{SG},D,1}-T_{0}+\frac{\mathrm{SpeedPara}\,\left(w_{\mathrm{SG},D,1}-w_{\mathrm{ref}}\right)}{2\,f_{0}\,\pi }}{T_{\mathrm{speed}}}$
      | Automatically generated on 2025-10-09 21:30:14 .
  State_w_SG_D_1_4fd49 : Inport
  State_T_m_SG_D_1_4e3cf : Inport  Port=2
  Add_5725c : Sum
  Add_a8cee : Sum
  Constant_-1_8a2a7 : Constant  Value=-1
  Constant_2.0_10424 : Constant  Value=2.0
  Constant_SpeedPara_3e6da : Constant  Value=SpeedPara
  Constant_T_0_36e72 : Constant  Value=T_0
  Constant_T_speed_d2b0e : Constant  Value=T_speed
  Constant_f0_1878c : Constant  Value=f0
  Constant_pi_d63a7 : Constant  Value=pi
  Constant_w_ref_cfdb4 : Constant  Value=w_ref
  Divide_b7672 : Product  Inputs=*/
  Divide_f3ea1 : Product  Inputs=*/
  Product_03024 : Product
  Product_04453 : Product
  Product_0f02d : Product
  Product_f7eb3 : Product
  Subtract_71d80 : Sum  Inputs=+-
  Blockout_d_T_m_SG_D_1_8a3f6 : Outport
  wires:
  Constant_-1_8a2a7/1 -> Product_04453/1
  Constant_w_ref_cfdb4/1 -> Add_a8cee/2
  State_w_SG_D_1_4fd49/1 -> Product_04453/2
  Add_5725c/1 -> Subtract_71d80/1
  Add_a8cee/1 -> Product_f7eb3/2
  Product_04453/1 -> Add_a8cee/1
  Constant_2.0_10424/1 -> Product_03024/1
  Constant_pi_d63a7/1 -> Product_03024/2
  Constant_SpeedPara_3e6da/1 -> Product_f7eb3/1
  Product_03024/1 -> Product_0f02d/1
  Constant_f0_1878c/1 -> Product_0f02d/2
  Constant_T_speed_d2b0e/1 -> Divide_b7672/2
  Product_f7eb3/1 -> Divide_f3ea1/1
  Product_0f02d/1 -> Divide_f3ea1/2
  Divide_f3ea1/1 -> Add_5725c/1
  Constant_T_0_36e72/1 -> Add_5725c/2
  State_T_m_SG_D_1_4e3cf/1 -> Subtract_71d80/2
  Subtract_71d80/1 -> Divide_b7672/1
  Divide_b7672/1 -> Blockout_d_T_m_SG_D_1_8a3f6/1

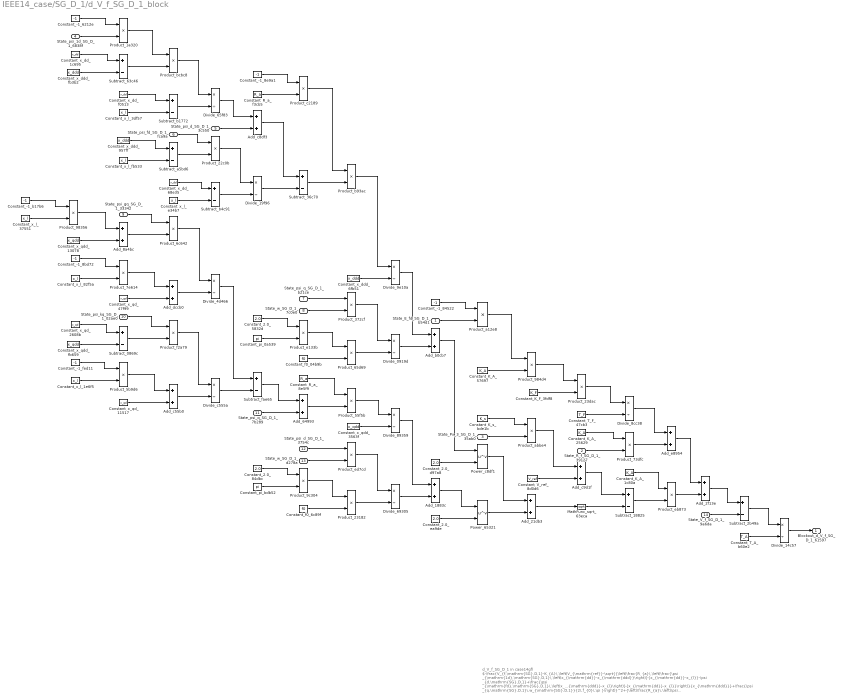
== system IEEE14_case/SG_D_1/d_V_f_SG_D_1_block ==
  note: d_V_f_SG_D_1 in case14gfl
      | $-\frac{V_{f,\mathrm{SG},D,1}-K_{A}\,\left(V_{\mathrm{ref}}-\sqrt{{\left(\frac{R_{a}\,\left(\frac{\psi _{\mathrm{1d},\mathrm{SG},D,1}\,\left(x_{\mathrm{dd}}-x_{\mathrm{ddd}}\right)}{x_{\mathrm{dd}}-x_{l}}-\psi _{d,\mathrm{SG},D,1}+\frac{\psi _{\mathrm{fd},\mathrm{SG},D,1}\,\left(x_{\mathrm{ddd}}-x_{l}\right)}{x_{\mathrm{dd}}-x_{l}}\right)}{x_{\mathrm{ddd}}}+\frac{\psi _{q,\mathrm{SG},D,1}\,w_{\mathrm{SG},D,1}}{2\,f_{0}\,\pi }\right)}^2+{\left(\frac{R_{a}\,\left(\psi _{q,\mathrm{SG},D,1}+\frac{\psi _{\mathrm{gq},\mathrm{SG},D,1}\,\left(x_{l}-x_{\mathrm{qdd}}\right)}{x_{l}-x_{\mathrm{qd}}}+\frac{\psi _{\mathrm{kq},\mathrm{SG},D,1}\,\left(x_{\mathrm{qd}}-x_{\mathrm{qdd}}\right)}{x_{l}-x_{\mathrm{qd}}}\right)}{x_{\mathrm{qdd}}}+\frac{\psi _{d,\mathrm{SG},D,1}\,w_{\mathrm{SG},D,1}}{2\,f_{0}\,\pi }\right)}^2}+K_{s}\,\mathrm{Px}_{3,\mathrm{SG},D,1}\right)-K_{A}\,R_{f,\mathrm{SG},D,1}+\frac{E_{\mathrm{fd},\mathrm{SG},D,1}\,K_{A}\,K_{F}}{T_{F}}}{T_{A}}$
      | Automatically generated on 2025-10-09 21:30:20 .
  State_E_fd_SG_D_1_b54d1 : Inport
  State_R_f_SG_D_1_39127 : Inport  Port=2
  State_Px_3_SG_D_1_35ab0 : Inport  Port=3
  State_psi_1d_SG_D_1_6838f : Inport  Port=4
  State_psi_d_SG_D_1_3c550 : Inport  Port=5
  State_psi_fd_SG_D_1_fca9a : Inport  Port=6
  State_psi_q_SG_D_1_b21ce : Inport  Port=7
  State_w_SG_D_1_7c0e0 : Inport  Port=8
  State_psi_gq_SG_D_1_33342 : Inport  Port=9
  State_psi_kq_SG_D_1_02ae0 : Inport  Port=10
  State_psi_q_SG_D_1_7b289 : Inport  Port=11
  State_psi_d_SG_D_1_3754c : Inport  Port=12
  State_w_SG_D_1_d278a : Inport  Port=13
  State_V_f_SG_D_1_9a6da : Inport  Port=14
  Add_1883c : Sum
  Add_21db3 : Sum
  Add_2f13e : Sum
  Add_64993 : Sum
  Add_8a4bc : Sum
  Add_b0cb7 : Sum
  Add_c55b0 : Sum
  Add_c8df3 : Sum
  Add_c9d1f : Sum
  Add_dccb0 : Sum
  Add_e8954 : Sum
  Constant_-1_6212e : Constant  Value=-1
  Constant_-1_84522 : Constant  Value=-1
  Constant_-1_8bd72 : Constant  Value=-1
  Constant_-1_8e9a1 : Constant  Value=-1
  Constant_-1_b17b6 : Constant  Value=-1
  Constant_-1_fed11 : Constant  Value=-1
  Constant_2.0_5832d : Constant  Value=2.0
  Constant_2.0_84dbc : Constant  Value=2.0
  Constant_2.0_d97a8 : Constant  Value=2.0
  Constant_2.0_ea9de : Constant  Value=2.0
  Constant_K_A_1c80a : Constant  Value=K_A
  Constant_K_A_25629 : Constant  Value=K_A
  Constant_K_A_57697 : Constant  Value=K_A
  Constant_K_F_3fdf8 : Constant  Value=K_F
  Constant_K_s_bde1b : Constant  Value=K_s
  Constant_R_a_8e5f9 : Constant  Value=R_a
  Constant_R_a_f3cb5 : Constant  Value=R_a
  Constant_T_A_b60e2 : Constant  Value=T_A
  Constant_T_F_47cb3 : Constant  Value=T_F
  Constant_V_ref_8d0d6 : Constant  Value=V_ref
  Constant_f0_04b9b : Constant  Value=f0
  Constant_f0_6c89f : Constant  Value=f0
  Constant_pi_0a539 : Constant  Value=pi
  Constant_pi_bdb52 : Constant  Value=pi
  Constant_x_dd_1c695 : Constant  Value=x_dd
  Constant_x_dd_68e35 : Constant  Value=x_dd
  Constant_x_dd_f0513 : Constant  Value=x_dd
  Constant_x_ddd_6fb51 : Constant  Value=x_ddd
  Constant_x_ddd_957ff : Constant  Value=x_ddd
  Constant_x_ddd_fb3b2 : Constant  Value=x_ddd
  Constant_x_l_1e6f5 : Constant  Value=x_l
  Constant_x_l_37551 : Constant  Value=x_l
  Constant_x_l_3df57 : Constant  Value=x_l
  Constant_x_l_82f5a : Constant  Value=x_l
  Constant_x_l_e34b7 : Constant  Value=x_l
  Constant_x_l_fb533 : Constant  Value=x_l
  Constant_x_qd_11517 : Constant  Value=x_qd
  Constant_x_qd_2608b : Constant  Value=x_qd
  Constant_x_qd_47f99 : Constant  Value=x_qd
  Constant_x_qdd_13078 : Constant  Value=x_qdd
  Constant_x_qdd_3563f : Constant  Value=x_qdd
  Constant_x_qdd_fb659 : Constant  Value=x_qdd
  Divide_0919d : Product  Inputs=*/
  Divide_14c57 : Product  Inputs=*/
  Divide_19f96 : Product  Inputs=*/
  Divide_4d466 : Product  Inputs=*/
  Divide_65f83 : Product  Inputs=*/
  Divide_69305 : Product  Inputs=*/
  Divide_89359 : Product  Inputs=*/
  Divide_8cc38 : Product  Inputs=*/
  Divide_9e10a : Product  Inputs=*/
  Divide_c555a : Product  Inputs=*/
  MathFunc_sqrt_63eca : Sqrt
  Power_65321 : Math  Operator=pow
  Power_c8df1 : Math  Operator=pow
  Product_1a320 : Product
  Product_22c0b : Product
  Product_23182 : Product
  Product_23dac : Product
  Product_372cf : Product
  Product_55f5b : Product
  Product_5b9d6 : Product
  Product_65d69 : Product
  Product_6c642 : Product
  Product_73dfc : Product
  Product_7e614 : Product
  Product_98356 : Product
  Product_984d4 : Product
  Product_9c304 : Product
  Product_a12e8 : Product
  Product_abbe4 : Product
  Product_b93ac : Product
  Product_bcbc8 : Product
  Product_c2189 : Product
  Product_e133b : Product
  Product_eb873 : Product
  Product_ed7cd : Product
  Product_f2a79 : Product
  Subtract_0869c : Sum  Inputs=+-
  Subtract_18825 : Sum  Inputs=+-
  Subtract_2b49a : Sum  Inputs=+-
  Subtract_36c70 : Sum  Inputs=+-
  Subtract_63c46 : Sum  Inputs=+-
  Subtract_a5bd6 : Sum  Inputs=+-
  Subtract_b1772 : Sum  Inputs=+-
  Subtract_b4c91 : Sum  Inputs=+-
  Subtract_fae65 : Sum  Inputs=+-
  Blockout_d_V_f_SG_D_1_61597 : Outport
  wires:
  Constant_-1_fed11/1 -> Product_5b9d6/1
  Constant_-1_b17b6/1 -> Product_98356/1
  State_psi_d_SG_D_1_3754c/1 -> Product_ed7cd/1
  Constant_x_qd_11517/1 -> Add_c55b0/2
  Constant_x_qdd_13078/1 -> Add_8a4bc/2
  State_w_SG_D_1_d278a/1 -> Product_ed7cd/2
  Constant_x_l_37551/1 -> Product_98356/2
  Subtract_36c70/1 -> Product_b93ac/2
  Constant_x_l_1e6f5/1 -> Product_5b9d6/2
  Constant_x_dd_1c695/1 -> Subtract_63c46/1
  Constant_R_a_f3cb5/1 -> Product_c2189/2
  Constant_-1_6212e/1 -> Product_1a320/1
  Divide_19f96/1 -> Subtract_36c70/2
  Constant_x_ddd_fb3b2/1 -> Subtract_63c46/2
  Add_c55b0/1 -> Divide_c555a/2
  State_psi_1d_SG_D_1_6838f/1 -> Product_1a320/2
  Add_dccb0/1 -> Divide_4d466/2
  Subtract_0869c/1 -> Product_f2a79/2
  Product_23dac/1 -> Divide_8cc38/1
  Product_e133b/1 -> Product_65d69/1
  Product_98356/1 -> Add_8a4bc/1
  Constant_-1_8bd72/1 -> Product_7e614/1
  Constant_x_l_82f5a/1 -> Product_7e614/2
  Add_c8df3/1 -> Subtract_36c70/1
  Constant_2.0_84dbc/1 -> Product_9c304/1
  Constant_x_qd_2608b/1 -> Subtract_0869c/1
  Product_1a320/1 -> Product_bcbc8/1
  Constant_pi_bdb52/1 -> Product_9c304/2
  Constant_x_qdd_fb659/1 -> Subtract_0869c/2
  Subtract_63c46/1 -> Product_bcbc8/2
  State_psi_q_SG_D_1_7b289/1 -> Add_64993/2
  Constant_x_dd_f0513/1 -> Subtract_b1772/1
  Constant_x_l_3df57/1 -> Subtract_b1772/2
  Constant_x_ddd_957ff/1 -> Subtract_a5bd6/1
  Constant_x_l_fb533/1 -> Subtract_a5bd6/2
  State_psi_gq_SG_D_1_33342/1 -> Product_6c642/1
  Add_8a4bc/1 -> Product_6c642/2
  Product_7e614/1 -> Add_dccb0/1
  Constant_x_qd_47f99/1 -> Add_dccb0/2
  Divide_65f83/1 -> Add_c8df3/1
  Subtract_b1772/1 -> Divide_65f83/2
  State_psi_kq_SG_D_1_02ae0/1 -> Product_f2a79/1
  Divide_14c57/1 -> Blockout_d_V_f_SG_D_1_61597/1
  Product_5b9d6/1 -> Add_c55b0/1
  Product_bcbc8/1 -> Divide_65f83/1
  State_psi_fd_SG_D_1_fca9a/1 -> Product_22c0b/1
  State_w_SG_D_1_7c0e0/1 -> Product_372cf/2
  Subtract_a5bd6/1 -> Product_22c0b/2
  Constant_x_dd_68e35/1 -> Subtract_b4c91/1
  Constant_x_l_e34b7/1 -> Subtract_b4c91/2
  Product_6c642/1 -> Divide_4d466/1
  Product_c2189/1 -> Product_b93ac/1
  Product_f2a79/1 -> Divide_c555a/1
  State_psi_d_SG_D_1_3c550/1 -> Add_c8df3/2
  Product_22c0b/1 -> Divide_19f96/1
  Subtract_b4c91/1 -> Divide_19f96/2
  Divide_4d466/1 -> Subtract_fae65/1
  Divide_c555a/1 -> Subtract_fae65/2
  Constant_-1_8e9a1/1 -> Product_c2189/1
  Constant_2.0_5832d/1 -> Product_e133b/1
  Constant_pi_0a539/1 -> Product_e133b/2
  Subtract_fae65/1 -> Add_64993/1
  State_psi_q_SG_D_1_b21ce/1 -> Product_372cf/1
  Constant_f0_04b9b/1 -> Product_65d69/2
  Constant_R_a_8e5f9/1 -> Product_55f5b/1
  Add_64993/1 -> Product_55f5b/2
  Product_9c304/1 -> Product_23182/1
  Power_c8df1/1 -> Add_21db3/1
  Constant_f0_6c89f/1 -> Product_23182/2
  Product_b93ac/1 -> Divide_9e10a/1
  Constant_x_ddd_6fb51/1 -> Divide_9e10a/2
  Product_372cf/1 -> Divide_0919d/1
  Product_65d69/1 -> Divide_0919d/2
  Product_55f5b/1 -> Divide_89359/1
  Constant_x_qdd_3563f/1 -> Divide_89359/2
  Product_ed7cd/1 -> Divide_69305/1
  Product_23182/1 -> Divide_69305/2
  Divide_9e10a/1 -> Add_b0cb7/1
  Divide_0919d/1 -> Add_b0cb7/2
  Divide_89359/1 -> Add_1883c/1
  Divide_69305/1 -> Add_1883c/2
  Constant_-1_84522/1 -> Product_a12e8/1
  State_E_fd_SG_D_1_b54d1/1 -> Product_a12e8/2
  Add_b0cb7/1 -> Power_c8df1/1
  Constant_2.0_d97a8/1 -> Power_c8df1/2
  Add_1883c/1 -> Power_65321/1
  Constant_2.0_ea9de/1 -> Power_65321/2
  Product_a12e8/1 -> Product_984d4/1
  Constant_K_A_57697/1 -> Product_984d4/2
  Constant_K_s_bde1b/1 -> Product_abbe4/1
  State_Px_3_SG_D_1_35ab0/1 -> Product_abbe4/2
  Power_65321/1 -> Add_21db3/2
  Divide_8cc38/1 -> Add_e8954/1
  Product_984d4/1 -> Product_23dac/1
  Constant_K_F_3fdf8/1 -> Product_23dac/2
  Product_abbe4/1 -> Add_c9d1f/1
  Constant_V_ref_8d0d6/1 -> Add_c9d1f/2
  Add_21db3/1 -> MathFunc_sqrt_63eca/1
  Constant_T_F_47cb3/1 -> Divide_8cc38/2
  Constant_K_A_25629/1 -> Product_73dfc/1
  State_R_f_SG_D_1_39127/1 -> Product_73dfc/2
  Add_c9d1f/1 -> Subtract_18825/1
  MathFunc_sqrt_63eca/1 -> Subtract_18825/2
  Constant_T_A_b60e2/1 -> Divide_14c57/2
  Product_73dfc/1 -> Add_e8954/2
  Constant_K_A_1c80a/1 -> Product_eb873/1
  Subtract_18825/1 -> Product_eb873/2
  Add_e8954/1 -> Add_2f13e/1
  Product_eb873/1 -> Add_2f13e/2
  Add_2f13e/1 -> Subtract_2b49a/1
  State_V_f_SG_D_1_9a6da/1 -> Subtract_2b49a/2
  Subtract_2b49a/1 -> Divide_14c57/1

== system IEEE14_case/SG_D_1/d_psi_1d_SG_D_1_block ==
  note: d_psi_1d_SG_D_1 in case14gfl
      | $-\frac{\psi _{\mathrm{1d},\mathrm{SG},D,1}-\psi _{\mathrm{fd},\mathrm{SG},D,1}+\frac{\left(x_{\mathrm{dd}}-x_{l}\right)\,\left(\frac{\psi _{\mathrm{1d},\mathrm{SG},D,1}\,\left(x_{\mathrm{dd}}-x_{\mathrm{ddd}}\right)}{x_{\mathrm{dd}}-x_{l}}-\psi _{d,\mathrm{SG},D,1}+\frac{\psi _{\mathrm{fd},\mathrm{SG},D,1}\,\left(x_{\mathrm{ddd}}-x_{l}\right)}{x_{\mathrm{dd}}-x_{l}}\right)}{x_{\mathrm{ddd}}}}{T_{\mathrm{ddd}}}$
      | Automatically generated on 2025-10-09 21:29:58 .
  State_psi_1d_SG_D_1_959f0 : Inport
  State_psi_fd_SG_D_1_00af5 : Inport  Port=2
  State_psi_1d_SG_D_1_c5f75 : Inport  Port=3
  State_psi_d_SG_D_1_719b4 : Inport  Port=4
  State_psi_fd_SG_D_1_15435 : Inport  Port=5
  Add_01ac5 : Sum
  Add_c64fe : Sum
  Add_e25a2 : Sum
  Constant_-1_073cc : Constant  Value=-1
  Constant_-1_4f936 : Constant  Value=-1
  Constant_T_ddd_84dc4 : Constant  Value=T_ddd
  Constant_x_dd_17125 : Constant  Value=x_dd
  Constant_x_dd_6e027 : Constant  Value=x_dd
  Constant_x_dd_afc17 : Constant  Value=x_dd
  Constant_x_dd_e9e56 : Constant  Value=x_dd
  Constant_x_ddd_0d45e : Constant  Value=x_ddd
  Constant_x_ddd_745ec : Constant  Value=x_ddd
  Constant_x_ddd_b55fe : Constant  Value=x_ddd
  Constant_x_l_7657e : Constant  Value=x_l
  Constant_x_l_c6670 : Constant  Value=x_l
  Constant_x_l_cbd05 : Constant  Value=x_l
  Constant_x_l_e26c2 : Constant  Value=x_l
  Divide_4a35b : Product  Inputs=*/
  Divide_cd9ce : Product  Inputs=*/
  Divide_de6af : Product  Inputs=*/
  Divide_eb1e2 : Product  Inputs=*/
  Product_261c0 : Product
  Product_62901 : Product
  Product_bb017 : Product
  Product_d1838 : Product
  Product_ea0dd : Product
  Subtract_1b9d0 : Sum  Inputs=+-
  Subtract_5055d : Sum  Inputs=+-
  Subtract_94f9a : Sum  Inputs=+-
  Subtract_ddda7 : Sum  Inputs=+-
  Subtract_e8729 : Sum  Inputs=+-
  Subtract_f31f6 : Sum  Inputs=+-
  Blockout_d_psi_1d_SG_D_1_ce82a : Outport
  wires:
  Product_ea0dd/1 -> Product_261c0/1
  Constant_-1_073cc/1 -> Product_ea0dd/1
  Subtract_ddda7/1 -> Product_261c0/2
  State_psi_1d_SG_D_1_c5f75/1 -> Product_ea0dd/2
  Subtract_94f9a/1 -> Product_bb017/1
  State_psi_d_SG_D_1_719b4/1 -> Add_01ac5/2
  Constant_x_dd_17125/1 -> Subtract_1b9d0/1
  Constant_x_l_7657e/1 -> Subtract_94f9a/2
  Constant_x_dd_e9e56/1 -> Subtract_ddda7/1
  Subtract_f31f6/1 -> Product_62901/2
  Constant_x_l_cbd05/1 -> Subtract_1b9d0/2
  Divide_de6af/1 -> Subtract_5055d/2
  Constant_x_ddd_b55fe/1 -> Subtract_ddda7/2
  Constant_x_ddd_0d45e/1 -> Subtract_f31f6/1
  Constant_x_l_e26c2/1 -> Subtract_f31f6/2
  Add_e25a2/1 -> Add_c64fe/1
  Product_261c0/1 -> Divide_4a35b/1
  Divide_eb1e2/1 -> Add_c64fe/2
  Subtract_1b9d0/1 -> Divide_4a35b/2
  State_psi_fd_SG_D_1_15435/1 -> Product_62901/1
  Constant_x_dd_afc17/1 -> Subtract_e8729/1
  Constant_x_l_c6670/1 -> Subtract_e8729/2
  Constant_x_ddd_745ec/1 -> Divide_eb1e2/2
  Subtract_5055d/1 -> Product_bb017/2
  Divide_4a35b/1 -> Add_01ac5/1
  Product_62901/1 -> Divide_de6af/1
  Subtract_e8729/1 -> Divide_de6af/2
  Product_bb017/1 -> Divide_eb1e2/1
  Constant_x_dd_6e027/1 -> Subtract_94f9a/1
  Add_01ac5/1 -> Subtract_5055d/1
  Constant_-1_4f936/1 -> Product_d1838/1
  State_psi_1d_SG_D_1_959f0/1 -> Product_d1838/2
  Product_d1838/1 -> Add_e25a2/1
  State_psi_fd_SG_D_1_00af5/1 -> Add_e25a2/2
  Add_c64fe/1 -> Divide_cd9ce/1
  Constant_T_ddd_84dc4/1 -> Divide_cd9ce/2
  Divide_cd9ce/1 -> Blockout_d_psi_1d_SG_D_1_ce82a/1
